simulink model "MIL_ASW"  (R2019b)
settings: Solver=FixedStepDiscrete  StartTime=0.0  StopTime=2  FixedStep=0.001  RelTol=1e-3  EnableMultiTasking=on
model workspace (MAT data in the model file):
  AccPedlCanVal : Simulink.Signal (value not decoded)
  AccPedlVal : Simulink.Signal (value not decoded)
  BrkPedlCanVal : Simulink.Signal (value not decoded)
  BrkPedlVal : Simulink.Signal (value not decoded)
  Cal1 : Simulink.Parameter (value not decoded)
  Cal10 : Simulink.Parameter (value not decoded)
  Cal11 : Simulink.Parameter (value not decoded)
  Cal12 : Simulink.Parameter (value not decoded)
  Cal2 : Simulink.Parameter (value not decoded)
  Cal3 : Simulink.Parameter (value not decoded)
  Cal4 : Simulink.Parameter (value not decoded)
  Cal5 : Simulink.Parameter (value not decoded)
  Cal6 : Simulink.Parameter (value not decoded)
  Cal7 : Simulink.Parameter (value not decoded)
  Cal8 : Simulink.Parameter (value not decoded)
  Cal9 : Simulink.Parameter (value not decoded)
  Clu1Act : Simulink.Signal (value not decoded)
  Clu1PTar : Simulink.Signal (value not decoded)
  Clu1Req : Simulink.Signal (value not decoded)
  Clu1TqTar : Simulink.Signal (value not decoded)
  Clu2Act : Simulink.Signal (value not decoded)
  Clu2PTar : Simulink.Signal (value not decoded)
  Clu2Req : Simulink.Signal (value not decoded)
  Clu2TqTar : Simulink.Signal (value not decoded)
  CluKissPtPLnch : Simulink.Parameter (value not decoded)
  CluOilTRawVal : Simulink.Signal (value not decoded)
  CluOilTVal : Simulink.Signal (value not decoded)
  CluOpenTqRatMax : Simulink.Parameter (value not decoded)
  CluPMap : Simulink.Parameter (value not decoded)
  CluPMax : Simulink.Parameter (value not decoded)
  CluPMaxGear1 : Simulink.Parameter (value not decoded)
  CluPMaxGear2 : Simulink.Parameter (value not decoded)
  CluPMaxGear3 : Simulink.Parameter (value not decoded)
  CluPMaxGear4 : Simulink.Parameter (value not decoded)
  CluPMaxGear5 : Simulink.Parameter (value not decoded)
  CluPMaxGear6 : Simulink.Parameter (value not decoded)
  CluPMaxGearR : Simulink.Parameter (value not decoded)
  CluPMin : Simulink.Parameter (value not decoded)
  CluPosnMax : Simulink.Parameter (value not decoded)
  CluSoln1IRawVal : Simulink.Signal (value not decoded)
  CluSoln1IReq : Simulink.Signal (value not decoded)
  CluSoln1IReqFlg : Simulink.Signal (value not decoded)
  CluSoln1IVal : Simulink.Signal (value not decoded)
  CluSoln1LineI : Simulink.Parameter (value not decoded)
  CluSoln1LineP : Simulink.Parameter (value not decoded)
  CluSoln1Pwm : Simulink.Signal (value not decoded)
  CluSoln2IRawVal : Simulink.Signal (value not decoded)
  CluSoln2IReq : Simulink.Signal (value not decoded)
  CluSoln2IReqFlg : Simulink.Signal (value not decoded)
  CluSoln2IVal : Simulink.Signal (value not decoded)
  CluSoln2LineI : Simulink.Parameter (value not decoded)
  CluSoln2LineP : Simulink.Parameter (value not decoded)
  CluSoln2Pwm : Simulink.Signal (value not decoded)
  CluTqMap : Simulink.Parameter (value not decoded)
  CrnkSpdRawVal : Simulink.Signal (value not decoded)
  CrnkSpdVal : Simulink.Signal (value not decoded)
  Drive_Intensity_Fuzzy : object (value not decoded)
  DrvIntenFzzy : Simulink.LookupTable (value not decoded)
  EngNIdle : Simulink.Parameter (value not decoded)
  EngNIdleMin : Simulink.Parameter (value not decoded)
  EngSpdCanVal : Simulink.Signal (value not decoded)
  EngThrCanVal : Simulink.Signal (value not decoded)
  EngTqAdd : Simulink.Parameter (value not decoded)
  EngTqCanVal : Simulink.Signal (value not decoded)
  EngTqIntvFlg : Simulink.Signal (value not decoded)
  EngTqIntvRat : Simulink.Signal (value not decoded)
  EngTqMapExtChartc : Simulink.Parameter (value not decoded)
  EngTqMapSpdIndx : Simulink.Parameter (value not decoded)
  EngTqMapThrtIndx : Simulink.Parameter (value not decoded)
  EngTqMapTqMax : Simulink.Parameter (value not decoded)
  EngTqMaxNorm : Simulink.Parameter (value not decoded)
  EngTqRef : Simulink.Parameter (value not decoded)
  EvenCluPRawVal : Simulink.Signal (value not decoded)
  EvenCluPVal : Simulink.Signal (value not decoded)
  EvenInpSpdRawVal : Simulink.Signal (value not decoded)
  EvenInpSpdVal : Simulink.Signal (value not decoded)
  FcnCallTime : Simulink.Parameter (value not decoded)
  FinalRat : Simulink.Parameter (value not decoded)
  Fork1A : Simulink.Parameter (value not decoded)
  Fork1Act : Simulink.Signal (value not decoded)
  Fork1B : Simulink.Parameter (value not decoded)
  Fork1DeltaSpdTar : Simulink.Parameter (value not decoded)
  Fork1MaxSpd1A : Simulink.Parameter (value not decoded)
  Fork1MaxSpd1B : Simulink.Parameter (value not decoded)
  Fork1MaxSpd2A : Simulink.Parameter (value not decoded)
  Fork1MaxSpd2B : Simulink.Parameter (value not decoded)
  Fork1PosnA : Simulink.Parameter (value not decoded)
  Fork1PosnB : Simulink.Parameter (value not decoded)
  Fork1PosnMaxSpd1A : Simulink.Parameter (value not decoded)
  Fork1PosnMaxSpd1B : Simulink.Parameter (value not decoded)
  Fork1PosnMaxSpd2A : Simulink.Parameter (value not decoded)
  Fork1PosnMaxSpd2B : Simulink.Parameter (value not decoded)
  Fork1PosnNeut : Simulink.Parameter (value not decoded)
  Fork1PosnNeutA : Simulink.Parameter (value not decoded)
  Fork1PosnNeutB : Simulink.Parameter (value not decoded)
  Fork1PosnRawVal : Simulink.Signal (value not decoded)
  Fork1PosnSyncA : Simulink.Parameter (value not decoded)
  Fork1PosnSyncB : Simulink.Parameter (value not decoded)
  Fork1PosnVal : Simulink.Signal (value not decoded)
  Fork1SyncTar : Simulink.Parameter (value not decoded)
  Fork2A : Simulink.Parameter (value not decoded)
  Fork2Act : Simulink.Signal (value not decoded)
  Fork2B : Simulink.Parameter (value not decoded)
  Fork2DeltaSpdTar : Simulink.Parameter (value not decoded)
  Fork2MaxSpd1A : Simulink.Parameter (value not decoded)
  Fork2MaxSpd1B : Simulink.Parameter (value not decoded)
  Fork2MaxSpd2A : Simulink.Parameter (value not decoded)
  Fork2MaxSpd2B : Simulink.Parameter (value not decoded)
  Fork2PosnA : Simulink.Parameter (value not decoded)
  Fork2PosnB : Simulink.Parameter (value not decoded)
  Fork2PosnMaxSpd1A : Simulink.Parameter (value not decoded)
  Fork2PosnMaxSpd1B : Simulink.Parameter (value not decoded)
  Fork2PosnMaxSpd2A : Simulink.Parameter (value not decoded)
  Fork2PosnMaxSpd2B : Simulink.Parameter (value not decoded)
  Fork2PosnNeut : Simulink.Parameter (value not decoded)
  Fork2PosnNeutA : Simulink.Parameter (value not decoded)
  Fork2PosnNeutB : Simulink.Parameter (value not decoded)
  Fork2PosnRawVal : Simulink.Signal (value not decoded)
  Fork2PosnSyncA : Simulink.Parameter (value not decoded)
  Fork2PosnSyncB : Simulink.Parameter (value not decoded)
  Fork2PosnVal : Simulink.Signal (value not decoded)
  Fork2SyncTar : Simulink.Parameter (value not decoded)
  Fork3A : Simulink.Parameter (value not decoded)
  Fork3Act : Simulink.Signal (value not decoded)
  Fork3B : Simulink.Parameter (value not decoded)
  Fork3DeltaSpdTar : Simulink.Parameter (value not decoded)
  Fork3MaxSpd1A : Simulink.Parameter (value not decoded)
  Fork3MaxSpd1B : Simulink.Parameter (value not decoded)
  Fork3MaxSpd2A : Simulink.Parameter (value not decoded)
  Fork3MaxSpd2B : Simulink.Parameter (value not decoded)
  Fork3PosnA : Simulink.Parameter (value not decoded)
  Fork3PosnB : Simulink.Parameter (value not decoded)
  Fork3PosnMaxSpd1A : Simulink.Parameter (value not decoded)
  Fork3PosnMaxSpd1B : Simulink.Parameter (value not decoded)
  Fork3PosnMaxSpd2A : Simulink.Parameter (value not decoded)
  Fork3PosnMaxSpd2B : Simulink.Parameter (value not decoded)
  Fork3PosnNeut : Simulink.Parameter (value not decoded)
  Fork3PosnNeutA : Simulink.Parameter (value not decoded)
  Fork3PosnNeutB : Simulink.Parameter (value not decoded)
  Fork3PosnRawVal : Simulink.Signal (value not decoded)
  Fork3PosnSyncA : Simulink.Parameter (value not decoded)
  Fork3PosnSyncB : Simulink.Parameter (value not decoded)
  Fork3PosnVal : Simulink.Signal (value not decoded)
  Fork3SyncTar : Simulink.Parameter (value not decoded)
  Fork4A : Simulink.Parameter (value not decoded)
  Fork4Act : Simulink.Signal (value not decoded)
  Fork4B : Simulink.Parameter (value not decoded)
  Fork4DeltaSpdTar : Simulink.Parameter (value not decoded)
  Fork4MaxSpd1A : Simulink.Parameter (value not decoded)
  Fork4MaxSpd1B : Simulink.Parameter (value not decoded)
  Fork4MaxSpd2A : Simulink.Parameter (value not decoded)
  Fork4MaxSpd2B : Simulink.Parameter (value not decoded)
  Fork4PosnA : Simulink.Parameter (value not decoded)
  Fork4PosnB : Simulink.Parameter (value not decoded)
  Fork4PosnMaxSpd1A : Simulink.Parameter (value not decoded)
  Fork4PosnMaxSpd1B : Simulink.Parameter (value not decoded)
  Fork4PosnMaxSpd2A : Simulink.Parameter (value not decoded)
  Fork4PosnMaxSpd2B : Simulink.Parameter (value not decoded)
  Fork4PosnNeut : Simulink.Parameter (value not decoded)
  Fork4PosnNeutA : Simulink.Parameter (value not decoded)
  Fork4PosnNeutB : Simulink.Parameter (value not decoded)
  Fork4PosnRawVal : Simulink.Signal (value not decoded)
  Fork4PosnSyncA : Simulink.Parameter (value not decoded)
  Fork4PosnSyncB : Simulink.Parameter (value not decoded)
  Fork4PosnVal : Simulink.Signal (value not decoded)
  Fork4SyncTar : Simulink.Parameter (value not decoded)
  FrntWhlRd : Simulink.Parameter (value not decoded)
  GearIdx : Simulink.Parameter (value not decoded)
  GearMax : Simulink.Parameter (value not decoded)
  GearRat : Simulink.Parameter (value not decoded)
  Launch_Engage_Fuzzy : object (value not decoded)
  LnchEngmtFzzy : Simulink.LookupTable (value not decoded)
  LubeSolnIRawVal : Simulink.Signal (value not decoded)
  LubeSolnIReq : Simulink.Signal (value not decoded)
  LubeSolnIVal : Simulink.Signal (value not decoded)
  LubeSolnLineI : Simulink.Parameter (value not decoded)
  LubeSolnLineP : Simulink.Parameter (value not decoded)
  LubeSolnPwm : Simulink.Signal (value not decoded)
  MaiLineSolnIRawVal : Simulink.Signal (value not decoded)
  MaiLineSolnIReq : Simulink.Signal (value not decoded)
  MaiLineSolnIVal : Simulink.Signal (value not decoded)
  MaiLineSolnLineI : Simulink.Parameter (value not decoded)
  MaiLineSolnLineP : Simulink.Parameter (value not decoded)
  MaiLineSolnPwm : Simulink.Signal (value not decoded)
  OddCluPRawVal : Simulink.Signal (value not decoded)
  OddCluPVal : Simulink.Signal (value not decoded)
  OddInpSpdRawVal : Simulink.Signal (value not decoded)
  OddInpSpdVal : Simulink.Signal (value not decoded)
  OutpSpdRawVal : Simulink.Signal (value not decoded)
  OutpSpdVal : Simulink.Signal (value not decoded)
  PsnsrLineP : Simulink.Parameter (value not decoded)
  PsnsrLineV : Simulink.Parameter (value not decoded)
  SftLvrCanVal : Simulink.Signal (value not decoded)
  SftLvrCfm : Simulink.Signal (value not decoded)
  SftLvrVal : Simulink.Signal (value not decoded)
  Shaft1GearAct : Simulink.Signal (value not decoded)
  Shaft1GearReq : Simulink.Signal (value not decoded)
  Shaft2GearAct : Simulink.Signal (value not decoded)
  Shaft2GearReq : Simulink.Signal (value not decoded)
  ShiftMux1SwtReq : Simulink.Signal (value not decoded)
  ShiftMux2SwtReq : Simulink.Signal (value not decoded)
  ShiftSdlEcoDwnSeln : Simulink.Parameter (value not decoded)
  ShiftSdlEcoDwnShift : Simulink.Parameter (value not decoded)
  ShiftSdlEcoUpSeln : Simulink.Parameter (value not decoded)
  ShiftSdlEcoUpShift : Simulink.Parameter (value not decoded)
  ShiftSdlPwrDwnSeln : Simulink.Parameter (value not decoded)
  ShiftSdlPwrDwnShift : Simulink.Parameter (value not decoded)
  ShiftSdlPwrUpSeln : Simulink.Parameter (value not decoded)
  ShiftSdlPwrUpShift : Simulink.Parameter (value not decoded)
  ShiftSdlSACDwnSeln : Simulink.Parameter (value not decoded)
  ShiftSdlSACDwnShift : Simulink.Parameter (value not decoded)
  ShiftSdlSACUpSeln : Simulink.Parameter (value not decoded)
  ShiftSdlSACUpShift : Simulink.Parameter (value not decoded)
  ShiftSdlThrPedlIdx : Simulink.Parameter (value not decoded)
  ShiftSoln1IRawVal : Simulink.Signal (value not decoded)
  ShiftSoln1IReq : Simulink.Signal (value not decoded)
  ShiftSoln1IVal : Simulink.Signal (value not decoded)
  ShiftSoln1LineI : Simulink.Parameter (value not decoded)
  ShiftSoln1LineP : Simulink.Parameter (value not decoded)
  ShiftSoln1Pwm : Simulink.Signal (value not decoded)
  ShiftSoln2IRawVal : Simulink.Signal (value not decoded)
  ShiftSoln2IReq : Simulink.Signal (value not decoded)
  ShiftSoln2IVal : Simulink.Signal (value not decoded)
  ShiftSoln2LineI : Simulink.Parameter (value not decoded)
  ShiftSoln2LineP : Simulink.Parameter (value not decoded)
  ShiftSoln2Pwm : Simulink.Signal (value not decoded)
  SolnOutpTRawVal : Simulink.Signal (value not decoded)
  SolnOutpTVal : Simulink.Signal (value not decoded)
  TSnsr1LineR : Simulink.Parameter (value not decoded)
  TSnsr2LineR : Simulink.Parameter (value not decoded)
  TrsmNrGearAct : Simulink.Signal (value not decoded)
  TrsmNrGearReq : Simulink.Signal (value not decoded)
  TrsmNrPreGearAct : Simulink.Signal (value not decoded)
  TrsmNrPreGearReq : Simulink.Signal (value not decoded)
  Tsnsr1LineT : Simulink.Parameter (value not decoded)
  Tsnsr2LineT : Simulink.Parameter (value not decoded)
  VehSpdCanVal : Simulink.Signal (value not decoded)
  VehSpdTrsmEstimd : Simulink.Signal (value not decoded)
  VehSpdVal : Simulink.Signal (value not decoded)
  VlvBodyTRawVal : Simulink.Signal (value not decoded)
  VlvBodyTVal : Simulink.Signal (value not decoded)
symbols that are objects in the model workspace (value not decoded): CluPMap, CluSoln1LineI, CluSoln1LineP, CluSoln2LineI, CluSoln2LineP, CluTqMap, EngNIdle, EngNIdleMin, EngTqMapThrtIndx, EngTqMapTqMax, EngTqMaxNorm, FcnCallTime, FinalRat, Fork1A, Fork1B, Fork1DeltaSpdTar, Fork1PosnA, Fork1PosnB, Fork1PosnMaxSpd1A, Fork1PosnMaxSpd1B, Fork1PosnMaxSpd2A, Fork1PosnMaxSpd2B, Fork1PosnNeut, Fork1PosnNeutA, Fork1PosnNeutB, Fork1PosnSyncA, Fork1PosnSyncB, Fork1SyncTar, Fork2A, Fork2B, Fork2DeltaSpdTar, Fork2PosnA, Fork2PosnB, Fork2PosnMaxSpd1A, Fork2PosnMaxSpd1B, Fork2PosnMaxSpd2A, Fork2PosnMaxSpd2B, Fork2PosnNeut, Fork2PosnNeutA, Fork2PosnNeutB, Fork2PosnSyncA, Fork2PosnSyncB, Fork2SyncTar, Fork3A, Fork3B, Fork3DeltaSpdTar, Fork3PosnA, Fork3PosnB, Fork3PosnMaxSpd1A, Fork3PosnMaxSpd1B, Fork3PosnMaxSpd2A, Fork3PosnMaxSpd2B, Fork3PosnNeut, Fork3PosnNeutA, Fork3PosnNeutB, Fork3PosnSyncA, Fork3PosnSyncB, Fork3SyncTar, Fork4A, Fork4B
undefined symbols (not defined in the file or in its folder): in1, out1
libraries: simulink x44, fuzblock x3
(part 5 of 10)

== system MIL_ASW/Application_Software_SHAW/ASW_GearPressureControl/Fork 3 ==
  ForkDirReq : Inport
  ForkSyncPha : Inport  Port=2
  ForkDeltaSpdReq : Inport  Port=3
  ForkPosnReq : Inport  Port=4
  ForkDeltaSpdAct : Inport  Port=5
  ForkPosnVal : Inport  Port=6
  Enable : EnablePort  StatesWhenEnabling=reset
  Abs : Abs  OutDataTypeStr=uint16
  Abs2 : Abs  OutDataTypeStr=uint16
  Add4 : Sum  Inputs=+-  OutDataTypeStr=int16
  Add6 : Sum  Inputs=+-  OutDataTypeStr=int16
  Compare To Constant : simulink/Logic and Bit Operations/Compare To Constant  relop===  const=2  OutDataTypeStr=boolean
  Compare To Constant1 : simulink/Logic and Bit Operations/Compare To Constant  relop===  const=1  OutDataTypeStr=boolean
  Compare To Constant2 : simulink/Logic and Bit Operations/Compare To Constant  relop===  const=3  OutDataTypeStr=boolean
  Compare To Constant3 : simulink/Logic and Bit Operations/Compare To Constant  relop===  const=2  OutDataTypeStr=boolean
  Compare To Constant4 : simulink/Logic and Bit Operations/Compare To Constant  relop===  const=4  OutDataTypeStr=boolean
  Constant : Constant  Value=150  OutDataTypeStr=uint16
  Gain : Gain  Gain=5  OutDataTypeStr=uint16
  Gain1 : Gain  OutDataTypeStr=uint16
  Logical Operator : Logic  Operator=OR  AllPortsSameDT=off  OutDataTypeStr=boolean
  Logical Operator1 : Logic  Operator=OR  AllPortsSameDT=off  OutDataTypeStr=boolean
  Saturation : Saturate  UpperLimit=300  LowerLimit=0  OutDataTypeStr=uint16
  Switch : Switch  Criteria=u2 > Threshold
  Switch1 : Switch  Criteria=u2 > Threshold
  Switch2 : Switch  Criteria=u2 > Threshold
  Terminator : Terminator
  ForkPReq : Outport  VectorParamsAs1DForOutWhenUnconnected=off
  wires:
  ForkPosnReq/1 -> Switch1/1, Switch2/1
  ForkDeltaSpdReq/1 -> Add6/1
  ForkDeltaSpdAct/1 -> Add6/2
  Add6/1 -> Abs2/1
  Add4/1 -> Abs/1
  Abs2/1 -> Gain1/1
  Compare To Constant/1 -> Switch/2
  ForkSyncPha/1 -> Compare To Constant/1
  Constant/1 -> Switch/1
  Gain/1 -> Switch/3
  ForkDirReq/1 -> Compare To Constant3/1, Compare To Constant1/1, Compare To Constant4/1, Compare To Constant2/1
  Compare To Constant1/1 -> Logical Operator/1
  Compare To Constant3/1 -> Logical Operator/2
  Compare To Constant2/1 -> Logical Operator1/1
  Compare To Constant4/1 -> Logical Operator1/2
  Logical Operator/1 -> Switch1/2
  ForkPosnVal/1 -> Switch2/3, Switch1/3
  Logical Operator1/1 -> Switch2/2
  Switch1/1 -> Add4/1
  Switch2/1 -> Add4/2
  Switch/1 -> Saturation/1
  Saturation/1 -> ForkPReq/1
  Gain1/1 -> Terminator/1
  Abs/1 -> Gain/1

== system MIL_ASW/Application_Software_SHAW/ASW_GearPressureControl/Fork 4 ==
  ForkDirReq : Inport
  ForkSyncPha : Inport  Port=2
  ForkDeltaSpdReq : Inport  Port=3
  ForkPosnReq : Inport  Port=4
  ForkDeltaSpdAct : Inport  Port=5
  ForkPosnVal : Inport  Port=6
  Enable : EnablePort  StatesWhenEnabling=reset
  Abs : Abs  OutDataTypeStr=uint16
  Abs2 : Abs  OutDataTypeStr=uint16
  Add4 : Sum  Inputs=+-  OutDataTypeStr=int16
  Add6 : Sum  Inputs=+-  OutDataTypeStr=int16
  Compare To Constant : simulink/Logic and Bit Operations/Compare To Constant  relop===  const=2  OutDataTypeStr=boolean
  Compare To Constant1 : simulink/Logic and Bit Operations/Compare To Constant  relop===  const=1  OutDataTypeStr=boolean
  Compare To Constant2 : simulink/Logic and Bit Operations/Compare To Constant  relop===  const=3  OutDataTypeStr=boolean
  Compare To Constant3 : simulink/Logic and Bit Operations/Compare To Constant  relop===  const=2  OutDataTypeStr=boolean
  Compare To Constant4 : simulink/Logic and Bit Operations/Compare To Constant  relop===  const=4  OutDataTypeStr=boolean
  Constant : Constant  Value=150  OutDataTypeStr=uint16
  Gain : Gain  Gain=5  OutDataTypeStr=uint16
  Gain1 : Gain  OutDataTypeStr=uint16
  Logical Operator : Logic  Operator=OR  AllPortsSameDT=off  OutDataTypeStr=boolean
  Logical Operator1 : Logic  Operator=OR  AllPortsSameDT=off  OutDataTypeStr=boolean
  Saturation : Saturate  UpperLimit=300  LowerLimit=0  OutDataTypeStr=uint16
  Switch : Switch  Criteria=u2 > Threshold
  Switch1 : Switch  Criteria=u2 > Threshold
  Switch2 : Switch  Criteria=u2 > Threshold
  Terminator : Terminator
  ForkPReq : Outport  VectorParamsAs1DForOutWhenUnconnected=off
  wires:
  Abs/1 -> Gain/1
  Gain1/1 -> Terminator/1
  Saturation/1 -> ForkPReq/1
  Switch/1 -> Saturation/1
  Switch2/1 -> Add4/2
  Switch1/1 -> Add4/1
  Logical Operator1/1 -> Switch2/2
  ForkPosnVal/1 -> Switch1/3, Switch2/3
  Logical Operator/1 -> Switch1/2
  Compare To Constant4/1 -> Logical Operator1/2
  Compare To Constant2/1 -> Logical Operator1/1
  Compare To Constant3/1 -> Logical Operator/2
  Compare To Constant1/1 -> Logical Operator/1
  ForkDirReq/1 -> Compare To Constant2/1, Compare To Constant4/1, Compare To Constant1/1, Compare To Constant3/1
  Gain/1 -> Switch/3
  Constant/1 -> Switch/1
  ForkSyncPha/1 -> Compare To Constant/1
  Compare To Constant/1 -> Switch/2
  Abs2/1 -> Gain1/1
  Add4/1 -> Abs/1
  Add6/1 -> Abs2/1
  ForkDeltaSpdAct/1 -> Add6/2
  ForkDeltaSpdReq/1 -> Add6/1
  ForkPosnReq/1 -> Switch2/1, Switch1/1

== system MIL_ASW/Application_Software_SHAW/ASW_GearPressureControl/PID ==
  In1 : Inport
  1/100 : Gain  Gain=1/100  OutDataTypeStr=uint16
  1/1000ms : Gain  Gain=1/1000  OutDataTypeStr=int32
  Add1 : Sum  Inputs=+-+  OutDataTypeStr=int16
  Add7 : Sum  Inputs=+-  OutDataTypeStr=int16
  Add8 : Sum  Inputs=+++  OutDataTypeStr=int32
  Add9 : Sum  OutDataTypeStr=int32
  Gain2 : Gain  Gain=1000/FcnCallTime  OutDataTypeStr=int32
  Gain3 : Gain  Gain=FcnCallTime  OutDataTypeStr=int32
  Gain4 : Gain  Gain=1000  OutDataTypeStr=int32
  Gain6 : Gain  Gain=2  OutDataTypeStr=int32
  Kd*100 : Gain  Gain=0  OutDataTypeStr=int32
  Ki*100 : Gain  Gain=100  OutDataTypeStr=int32
  Kp*100 : Gain  Gain=15  OutDataTypeStr=int32
  Memory{1..3,5} (4 alike) : Memory  InheritSampleTime=on
  Saturation1 : Saturate  UpperLimit=100000  LowerLimit=0  OutDataTypeStr=int32
  Saturation2 : Saturate  UpperLimit=30000  LowerLimit=-30000
  Out1 : Outport  VectorParamsAs1DForOutWhenUnconnected=off
  wires:
  Add7/1 -> Kp*100/1
  Saturation2/1 -> Add9/2
  Ki*100/1 -> Gain3/1
  Kp*100/1 -> Gain4/1
  Memory2/1 -> Add7/2
  Saturation1/1 -> 1/100/1, Memory3/1
  Add9/1 -> Saturation1/1
  Add8/1 -> 1/1000ms/1
  In1/1 -> Add7/1, Memory1/1, Add1/1, Ki*100/1, Memory2/1
  Gain3/1 -> Add8/2
  Gain4/1 -> Add8/1
  Memory3/1 -> Add9/1
  Add1/1 -> Kd*100/1
  Gain6/1 -> Add1/2
  Kd*100/1 -> Gain2/1
  Memory5/1 -> Add1/3
  Gain2/1 -> Add8/3
  Memory1/1 -> Memory5/1, Gain6/1
  1/1000ms/1 -> Saturation2/1
  1/100/1 -> Out1/1

== system MIL_ASW/Application_Software_SHAW/ASW_GearPressureControl/PID1 ==
  In1 : Inport
  1/100 : Gain  Gain=1/100  OutDataTypeStr=uint16
  1/1000ms : Gain  Gain=1/1000  OutDataTypeStr=int32
  Add1 : Sum  Inputs=+-+  OutDataTypeStr=int16
  Add7 : Sum  Inputs=+-  OutDataTypeStr=int16
  Add8 : Sum  Inputs=+++  OutDataTypeStr=int32
  Add9 : Sum  OutDataTypeStr=int32
  Gain2 : Gain  Gain=1000/FcnCallTime  OutDataTypeStr=int32
  Gain3 : Gain  Gain=FcnCallTime  OutDataTypeStr=int32
  Gain4 : Gain  Gain=1000  OutDataTypeStr=int32
  Gain6 : Gain  Gain=2  OutDataTypeStr=int32
  Kd*100 : Gain  Gain=0  OutDataTypeStr=int32
  Ki*100 : Gain  Gain=100  OutDataTypeStr=int32
  Kp*100 : Gain  Gain=15  OutDataTypeStr=int32
  Memory{1..3,5} (4 alike) : Memory  InheritSampleTime=on
  Saturation1 : Saturate  UpperLimit=100000  LowerLimit=0  OutDataTypeStr=int32
  Saturation2 : Saturate  UpperLimit=30000  LowerLimit=-30000
  Out1 : Outport  VectorParamsAs1DForOutWhenUnconnected=off
  wires:
  1/100/1 -> Out1/1
  1/1000ms/1 -> Saturation2/1
  Memory1/1 -> Gain6/1, Memory5/1
  Gain2/1 -> Add8/3
  Memory5/1 -> Add1/3
  Kd*100/1 -> Gain2/1
  Gain6/1 -> Add1/2
  Add1/1 -> Kd*100/1
  Memory3/1 -> Add9/1
  Gain4/1 -> Add8/1
  Gain3/1 -> Add8/2
  In1/1 -> Memory2/1, Ki*100/1, Add1/1, Memory1/1, Add7/1
  Add8/1 -> 1/1000ms/1
  Add9/1 -> Saturation1/1
  Saturation1/1 -> Memory3/1, 1/100/1
  Memory2/1 -> Add7/2
  Kp*100/1 -> Gain4/1
  Ki*100/1 -> Gain3/1
  Saturation2/1 -> Add9/2
  Add7/1 -> Kp*100/1

== system MIL_ASW/Application_Software_SHAW/ASW_Interface/Accelerator Pedal Value Process ==
  AccPedlCanVal : Inport
  BrkPedlVal : Inport  Port=2
  Constant : Constant  Value=0  OutDataTypeStr=uint8
  Gain : Gain  Gain=100/255  OutDataTypeStr=uint8
  Switch : Switch  Criteria=u2 > Threshold  OutDataTypeStr=uint8
  AccPedlVal : Outport  OutDataTypeStr=uint8  VectorParamsAs1DForOutWhenUnconnected=off
  wires:
  BrkPedlVal/1 -> Switch/2
  Switch/1 -> Gain/1
  Constant/1 -> Switch/1
  Gain/1 -> AccPedlVal/1
  AccPedlCanVal/1 -> Switch/3

== system MIL_ASW/Application_Software_SHAW/ASW_Interface/Brake Pedal Value Process ==
  BrkPedlCanVal : Inport
  Compare To Constant : simulink/Logic and Bit Operations/Compare To Constant  relop=>  const=30  OutDataTypeStr=uint8
  Gain : Gain  Gain=100/255  OutDataTypeStr=uint8
  BrkPedlVal : Outport  OutDataTypeStr=uint8  VectorParamsAs1DForOutWhenUnconnected=off
  BrkSig : Outport  Port=2  OutDataTypeStr=uint8  VectorParamsAs1DForOutWhenUnconnected=off
  wires:
  Gain/1 -> Compare To Constant/1, BrkPedlVal/1
  BrkPedlCanVal/1 -> Gain/1
  Compare To Constant/1 -> BrkSig/1

== system MIL_ASW/Application_Software_SHAW/ASW_Interface/Clutch Pressure Sensor Value Process ==
  OddCluPRawVal : Inport
  EvenCluPRawVal : Inport  Port=2
  1-D Lookup Table1 : Lookup_n-D  NumberOfTableDimensions=1  BreakpointsForDimension1=PsnsrLineV  Table=PsnsrLineP  TableDataTypeStr=Inherit: Inherit from 'Table data'  ExtrapMethod=Clip  UseLastTableValue=on  InternalRulePriority=Speed  OutDataTypeStr=Inherit: Inherit from 'Table data'  RndMeth=Simplest  InputSameDT=on
  1-D Lookup Table3 : Lookup_n-D  NumberOfTableDimensions=1  BreakpointsForDimension1=PsnsrLineV  Table=PsnsrLineP  TableDataTypeStr=Inherit: Inherit from 'Table data'  ExtrapMethod=Clip  UseLastTableValue=on  InternalRulePriority=Speed  OutDataTypeStr=Inherit: Inherit from 'Table data'  RndMeth=Simplest  InputSameDT=on
  Constant1 : Constant  Value=1023  OutDataTypeStr=uint16
  Constant2 : Constant  Value=1023  OutDataTypeStr=uint16
  Divide1 : Product  Inputs=*/  OutDataTypeStr=uint16
  Divide3 : Product  Inputs=*/  OutDataTypeStr=uint16
  Gain1 : Gain  Gain=5000  OutDataTypeStr=uint32
  Gain4 : Gain  Gain=5000  OutDataTypeStr=uint32
  OddCluPVal : Outport  VectorParamsAs1DForOutWhenUnconnected=off
  EvenCluPVal : Outport  Port=2  VectorParamsAs1DForOutWhenUnconnected=off
  wires:
  EvenCluPRawVal/1 -> Gain1/1
  1-D Lookup Table1/1 -> EvenCluPVal/1
  Gain4/1 -> Divide3/1
  Divide3/1 -> 1-D Lookup Table3/1  "mV"
  OddCluPRawVal/1 -> Gain4/1
  1-D Lookup Table3/1 -> OddCluPVal/1
  Constant2/1 -> Divide3/2
  Gain1/1 -> Divide1/1
  Divide1/1 -> 1-D Lookup Table1/1  "mV"
  Constant1/1 -> Divide1/2

== system MIL_ASW/Application_Software_SHAW/ASW_Interface/Engine Information from CAN bus ==
  EngThrCanVal : Inport
  EngSpdCanVal : Inport  Port=2
  EngTqCanVal : Inport  Port=3  OutDataTypeStr=uint16
  Constant : Constant  Value=84800  OutDataTypeStr=int32
  Constant1 : Constant  Value=0  OutDataTypeStr=int32
  Data Type Conversion : DataTypeConversion  OutDataTypeStr=uint16
  Gain : Gain  Gain=100/255  OutDataTypeStr=uint8
  Gain1 : Gain  Gain=1/4  ParamDataTypeStr=uint16  OutDataTypeStr=uint16
  Gain4 : Gain  Gain=100/2  OutDataTypeStr=int32
  MinMax : MinMax  Function=max  Inputs=2
  Subtract : Sum  Inputs=+-  OutDataTypeStr=int32
  EngThrVal : Outport  VectorParamsAs1DForOutWhenUnconnected=off
  EngSpdVal : Outport  Port=2  VectorParamsAs1DForOutWhenUnconnected=off
  EngTqVal : Outport  Port=3  VectorParamsAs1DForOutWhenUnconnected=off
  wires:
  EngSpdCanVal/1 -> Gain1/1
  EngTqCanVal/1 -> Gain4/1
  Gain4/1 -> Subtract/1
  EngThrCanVal/1 -> Gain/1
  Gain/1 -> EngThrVal/1
  Gain1/1 -> EngSpdVal/1
  Subtract/1 -> MinMax/1
  Constant/1 -> Subtract/2
  MinMax/1 -> Data Type Conversion/1
  Data Type Conversion/1 -> EngTqVal/1
  Constant1/1 -> MinMax/2

== system MIL_ASW/Application_Software_SHAW/ASW_Interface/Fork Position Sensor Value Process ==
  Fork1PosnRawVal : Inport
  Fork2PosnRawVal : Inport  Port=2
  Fork3PosnRawVal : Inport  Port=3
  Fork4PosnRawVal : Inport  Port=4
  Gain{1..4} (4 alike) : Gain  OutDataTypeStr=uint16
  Saturation{,1..3} (4 alike) : Saturate  UpperLimit=900  LowerLimit=100
  Fork1PosnVal : Outport  OutDataTypeStr=uint16  VectorParamsAs1DForOutWhenUnconnected=off
  Fork2PosnVal : Outport  Port=2  OutDataTypeStr=uint16  VectorParamsAs1DForOutWhenUnconnected=off
  Fork3PosnVal : Outport  Port=3  OutDataTypeStr=uint16  VectorParamsAs1DForOutWhenUnconnected=off
  Fork4PosnVal : Outport  Port=4  OutDataTypeStr=uint16  VectorParamsAs1DForOutWhenUnconnected=off
  wires:
  Fork1PosnRawVal/1 -> Gain4/1
  Gain4/1 -> Saturation/1
  Fork2PosnRawVal/1 -> Gain1/1
  Gain1/1 -> Saturation1/1
  Fork3PosnRawVal/1 -> Gain2/1
  Gain2/1 -> Saturation2/1
  Fork4PosnRawVal/1 -> Gain3/1
  Gain3/1 -> Saturation3/1
  Saturation/1 -> Fork1PosnVal/1
  Saturation1/1 -> Fork2PosnVal/1
  Saturation2/1 -> Fork3PosnVal/1
  Saturation3/1 -> Fork4PosnVal/1

== system MIL_ASW/Application_Software_SHAW/ASW_Interface/Shift Lever Value Process ==
  SftLvrCanVal : Inport
  Constant : Constant  Value=0  OutDataTypeStr=uint8
  Constant1 : Constant  OutDataTypeStr=uint8
  Constant2 : Constant  Value=2  OutDataTypeStr=uint8
  Constant3 : Constant  Value=3  OutDataTypeStr=uint8
  Constant4 : Constant  Value=2  OutDataTypeStr=uint8
  Multiport Switch : MultiPortSwitch  DataPortOrder=Specify indices  DataPortIndices={8,7,6,5}  DataPortForDefault=Additional data port  DiagnosticForDefault=Warning  OutDataTypeStr=uint8
  SftLvrVal : Outport  OutDataTypeStr=uint8  VectorParamsAs1DForOutWhenUnconnected=off
  wires:
  SftLvrCanVal/1 -> Multiport Switch/1
  Constant/1 -> Multiport Switch/2
  Constant1/1 -> Multiport Switch/3
  Constant2/1 -> Multiport Switch/4
  Constant3/1 -> Multiport Switch/5
  Constant4/1 -> Multiport Switch/6
  Multiport Switch/1 -> SftLvrVal/1

== system MIL_ASW/Application_Software_SHAW/ASW_Interface/Solenoid Current Value Process ==
  ShiftSoln1IRawVal : Inport
  ShiftSoln2IRawVal : Inport  Port=2
  MaiLineSolnIRawVal : Inport  Port=3
  LubeSolnIRawVal : Inport  Port=4
  CluSoln1IRawVal : Inport  Port=5
  CluSoln2IRawVal : Inport  Port=6
  Gain{,1..5} (6 alike) : Gain  Gain=1000/2*5/1023  OutDataTypeStr=uint16
  ShiftSoln1IVal : Outport  VectorParamsAs1DForOutWhenUnconnected=off
  ShiftSoln2IVal : Outport  Port=2  VectorParamsAs1DForOutWhenUnconnected=off
  MaiLineSolnIVal : Outport  Port=3  VectorParamsAs1DForOutWhenUnconnected=off
  LubeSolnIVal : Outport  Port=4  VectorParamsAs1DForOutWhenUnconnected=off
  CluSoln1IVal : Outport  Port=5  VectorParamsAs1DForOutWhenUnconnected=off
  CluSoln2IVal : Outport  Port=6  VectorParamsAs1DForOutWhenUnconnected=off
  wires:
  ShiftSoln1IRawVal/1 -> Gain/1
  Gain/1 -> ShiftSoln1IVal/1
  ShiftSoln2IRawVal/1 -> Gain1/1
  Gain1/1 -> ShiftSoln2IVal/1
  MaiLineSolnIRawVal/1 -> Gain2/1
  Gain2/1 -> MaiLineSolnIVal/1
  LubeSolnIRawVal/1 -> Gain3/1
  Gain3/1 -> LubeSolnIVal/1
  CluSoln1IRawVal/1 -> Gain4/1
  Gain4/1 -> CluSoln1IVal/1
  Gain5/1 -> CluSoln2IVal/1
  CluSoln2IRawVal/1 -> Gain5/1

== system MIL_ASW/Application_Software_SHAW/ASW_Interface/Speed Sensor Value Process ==
  CrnkSpdRawVal : Inport
  OddInpSpdRawVal : Inport  Port=2
  EvenInpSpdRawVal : Inport  Port=3
  OutpSpdRawVal : Inport  Port=4
  Constant : Constant  Value=2*314/100*FrntWhlRd/60*36/10  OutDataTypeStr=uint16
  Constant4 : Constant  Value=FinalRat(1)  OutDataTypeStr=uint16
  Divide4 : Product  Inputs=*/  OutDataTypeStr=uint16
  Gain : Gain  Gain=60/36  OutDataTypeStr=uint16
  Gain1 : Gain  Gain=60/36  OutDataTypeStr=uint16
  Gain2 : Gain  Gain=60/36  OutDataTypeStr=uint16
  Gain3 : Gain  Gain=60/18  OutDataTypeStr=uint16
  Gain4 : Gain  Gain=100  ParamDataTypeStr=uint16
  Product : Product  OutDataTypeStr=uint16
  Saturation : Saturate  UpperLimit=6800  LowerLimit=0
  Saturation1 : Saturate  UpperLimit=6800  LowerLimit=0
  Saturation2 : Saturate  UpperLimit=6800  LowerLimit=0
  Saturation3 : Saturate  UpperLimit=8940  LowerLimit=0
  CrnkSpdVal : Outport  VectorParamsAs1DForOutWhenUnconnected=off
  OddInpSpdVal : Outport  Port=2  VectorParamsAs1DForOutWhenUnconnected=off
  EvenInpSpdVal : Outport  Port=3  VectorParamsAs1DForOutWhenUnconnected=off
  OutpSpdVal : Outport  Port=4  VectorParamsAs1DForOutWhenUnconnected=off
  VehSpdTrsmEstimd : Outport  Port=5  VectorParamsAs1DForOutWhenUnconnected=off
  wires:
  CrnkSpdRawVal/1 -> Gain/1
  Gain/1 -> Saturation/1
  OddInpSpdRawVal/1 -> Gain1/1
  Gain1/1 -> Saturation1/1
  EvenInpSpdRawVal/1 -> Gain2/1
  Gain2/1 -> Saturation2/1
  OutpSpdRawVal/1 -> Gain3/1
  Divide4/1 -> Saturation3/1, Product/1
  Constant/1 -> Product/2
  Product/1 -> VehSpdTrsmEstimd/1
  Saturation/1 -> CrnkSpdVal/1
  Saturation1/1 -> OddInpSpdVal/1
  Saturation2/1 -> EvenInpSpdVal/1
  Saturation3/1 -> OutpSpdVal/1
  Constant4/1 -> Divide4/2
  Gain4/1 -> Divide4/1
  Gain3/1 -> Gain4/1

== system MIL_ASW/Application_Software_SHAW/ASW_Interface/Temperature Sensor Value Process ==
  CluOilTVal : Inport
  ValvBodyTRawVal : Inport  Port=2
  SolnOutpTRawVal : Inport  Port=3
  1-D Lookup Table1 : Lookup_n-D  NumberOfTableDimensions=1  BreakpointsForDimension1=TSnsr1LineR  Table=Tsnsr1LineT  TableDataTypeStr=Inherit: Inherit from 'Table data'  ExtrapMethod=Clip  UseLastTableValue=on  InternalRulePriority=Speed  OutDataTypeStr=Inherit: Inherit from 'Table data'  RndMeth=Simplest  InputSameDT=on
  1-D Lookup Table2 : Lookup_n-D  NumberOfTableDimensions=1  BreakpointsForDimension1=TSnsr2LineR  Table=Tsnsr2LineT  TableDataTypeStr=Inherit: Inherit from 'Table data'  ExtrapMethod=Clip  UseLastTableValue=on  InternalRulePriority=Speed  OutDataTypeStr=Inherit: Inherit from 'Table data'  RndMeth=Simplest  InputSameDT=on
  1-D Lookup Table3 : Lookup_n-D  NumberOfTableDimensions=1  BreakpointsForDimension1=TSnsr1LineR  Table=Tsnsr1LineT  TableDataTypeStr=Inherit: Inherit from 'Table data'  ExtrapMethod=Clip  UseLastTableValue=on  InternalRulePriority=Speed  OutDataTypeStr=Inherit: Inherit from 'Table data'  RndMeth=Simplest  InputSameDT=on
  Add1 : Sum  Inputs=-+
  Add2 : Sum  Inputs=-+
  Add3 : Sum  Inputs=-+
  Constant1 : Constant  Value=1023  OutDataTypeStr=uint16
  Constant2 : Constant  Value=1023  OutDataTypeStr=uint16
  Constant3 : Constant  Value=1023  OutDataTypeStr=uint16
  Divide1 : Product  Inputs=*/  OutDataTypeStr=uint16
  Divide2 : Product  Inputs=*/  OutDataTypeStr=uint16
  Divide3 : Product  Inputs=*/  OutDataTypeStr=uint16
  Gain : Gain  Gain=2600  OutDataTypeStr=uint32
  Gain1 : Gain  Gain=510  OutDataTypeStr=uint32
  Gain2 : Gain  Gain=2600  OutDataTypeStr=uint32
  CluOilTRawVal : Outport  VectorParamsAs1DForOutWhenUnconnected=off
  ValvBodyTVal : Outport  Port=2  VectorParamsAs1DForOutWhenUnconnected=off
  SolnOutpTVal : Outport  Port=3  VectorParamsAs1DForOutWhenUnconnected=off
  wires:
  Gain/1 -> Divide3/1
  Constant1/1 -> Add3/2
  Add3/1 -> Divide3/2
  Divide3/1 -> 1-D Lookup Table3/1  "R"
  CluOilTVal/1 -> Add3/1, Gain/1
  1-D Lookup Table3/1 -> CluOilTRawVal/1
  Divide2/1 -> 1-D Lookup Table2/1  "10R"
  1-D Lookup Table2/1 -> SolnOutpTVal/1
  Gain2/1 -> Divide1/1
  Constant3/1 -> Add2/2
  Add2/1 -> Divide1/2
  Divide1/1 -> 1-D Lookup Table1/1  "R"
  ValvBodyTRawVal/1 -> Gain2/1, Add2/1
  1-D Lookup Table1/1 -> ValvBodyTVal/1
  Gain1/1 -> Divide2/1
  Constant2/1 -> Add1/2
  Add1/1 -> Divide2/2
  SolnOutpTRawVal/1 -> Add1/1, Gain1/1

== system MIL_ASW/Application_Software_SHAW/ASW_Interface/Vehicle Speed Value Process ==
  VehSpdCanVal : Inport
  Gain : Gain  Gain=100/64  OutDataTypeStr=uint16
  VehSpdVal : Outport  VectorParamsAs1DForOutWhenUnconnected=off
  wires:
  VehSpdCanVal/1 -> Gain/1
  Gain/1 -> VehSpdVal/1

== system MIL_ASW/Application_Software_SHAW/ASW_MainLineControl/PID ==
  In1 : Inport
  1/100 : Gain  Gain=1/100  OutDataTypeStr=uint16
  1/1000ms : Gain  Gain=1/1000  OutDataTypeStr=int32
  Add1 : Sum  Inputs=+-+  OutDataTypeStr=int16
  Add7 : Sum  Inputs=+-  OutDataTypeStr=int16
  Add8 : Sum  Inputs=+++  OutDataTypeStr=int32
  Add9 : Sum  OutDataTypeStr=int32
  Gain2 : Gain  Gain=1000/FcnCallTime  OutDataTypeStr=int32
  Gain3 : Gain  Gain=FcnCallTime  OutDataTypeStr=int32
  Gain4 : Gain  Gain=1000  OutDataTypeStr=int32
  Gain6 : Gain  Gain=2  OutDataTypeStr=int32
  Kd*100 : Gain  Gain=0  OutDataTypeStr=int32
  Ki*100 : Gain  Gain=100  OutDataTypeStr=int32
  Kp*100 : Gain  Gain=15  OutDataTypeStr=int32
  Memory{1..3,5} (4 alike) : Memory  InheritSampleTime=on
  Saturation1 : Saturate  UpperLimit=100000  LowerLimit=0  OutDataTypeStr=int32
  Saturation2 : Saturate  UpperLimit=30000  LowerLimit=-30000
  Out1 : Outport  VectorParamsAs1DForOutWhenUnconnected=off
  wires:
  Add7/1 -> Kp*100/1
  Saturation2/1 -> Add9/2
  Ki*100/1 -> Gain3/1
  Kp*100/1 -> Gain4/1
  Memory2/1 -> Add7/2
  Saturation1/1 -> 1/100/1, Memory3/1
  Add9/1 -> Saturation1/1
  Add8/1 -> 1/1000ms/1
  In1/1 -> Add7/1, Memory1/1, Add1/1, Ki*100/1, Memory2/1
  Gain3/1 -> Add8/2
  Gain4/1 -> Add8/1
  Memory3/1 -> Add9/1
  Add1/1 -> Kd*100/1
  Gain6/1 -> Add1/2
  Kd*100/1 -> Gain2/1
  Memory5/1 -> Add1/3
  Gain2/1 -> Add8/3
  Memory1/1 -> Memory5/1, Gain6/1
  1/1000ms/1 -> Saturation2/1
  1/100/1 -> Out1/1

== system MIL_ASW/Application_Software_SHAW/ASW_MainLineControl/PID1 ==
  In1 : Inport
  1/100 : Gain  Gain=1/100  OutDataTypeStr=uint16
  1/1000ms : Gain  Gain=1/1000  OutDataTypeStr=int32
  Add1 : Sum  Inputs=+-+  OutDataTypeStr=int16
  Add7 : Sum  Inputs=+-  OutDataTypeStr=int16
  Add8 : Sum  Inputs=+++  OutDataTypeStr=int32
  Add9 : Sum  OutDataTypeStr=int32
  Gain2 : Gain  Gain=1000/FcnCallTime  OutDataTypeStr=int32
  Gain3 : Gain  Gain=FcnCallTime  OutDataTypeStr=int32
  Gain4 : Gain  Gain=1000  OutDataTypeStr=int32
  Gain6 : Gain  Gain=2  OutDataTypeStr=int32
  Kd*100 : Gain  Gain=0  OutDataTypeStr=int32
  Ki*100 : Gain  Gain=100  OutDataTypeStr=int32
  Kp*100 : Gain  Gain=15  OutDataTypeStr=int32
  Memory{1..3,5} (4 alike) : Memory  InheritSampleTime=on
  Saturation1 : Saturate  UpperLimit=100000  LowerLimit=0  OutDataTypeStr=int32
  Saturation2 : Saturate  UpperLimit=30000  LowerLimit=-30000
  Out1 : Outport  VectorParamsAs1DForOutWhenUnconnected=off
  wires:
  Add7/1 -> Kp*100/1
  Saturation2/1 -> Add9/2
  Ki*100/1 -> Gain3/1
  Kp*100/1 -> Gain4/1
  Memory2/1 -> Add7/2
  Saturation1/1 -> 1/100/1, Memory3/1
  Add9/1 -> Saturation1/1
  Add8/1 -> 1/1000ms/1
  In1/1 -> Add7/1, Memory1/1, Add1/1, Ki*100/1, Memory2/1
  Gain3/1 -> Add8/2
  Gain4/1 -> Add8/1
  Memory3/1 -> Add9/1
  Add1/1 -> Kd*100/1
  Gain6/1 -> Add1/2
  Kd*100/1 -> Gain2/1
  Memory5/1 -> Add1/3
  Gain2/1 -> Add8/3
  Memory1/1 -> Memory5/1, Gain6/1
  1/1000ms/1 -> Saturation2/1
  1/100/1 -> Out1/1

== system MIL_ASW/Application_Software_SHAW/ASW_ShaftAccessControl/Shift lever match to gear ==
  SftLvrVal : Inport
  TrsmNrGearAct : Inport  Port=2
  TrsmNrPreGearAct : Inport  Port=3
  Shift lever confirm logic : Stateflow chart  TreatAsAtomicUnit=on
  SftLvrCfm : Outport  VectorParamsAs1DForOutWhenUnconnected=off
  wires:
  TrsmNrPreGearAct/1 -> Shift lever confirm logic/3(PreGearRx)
  SftLvrVal/1 -> Shift lever confirm logic/1(ShiftLvrRx)
  TrsmNrGearAct/1 -> Shift lever confirm logic/2(GearRx)
  Shift lever confirm logic/1(SftLvrCfm) -> SftLvrCfm/1

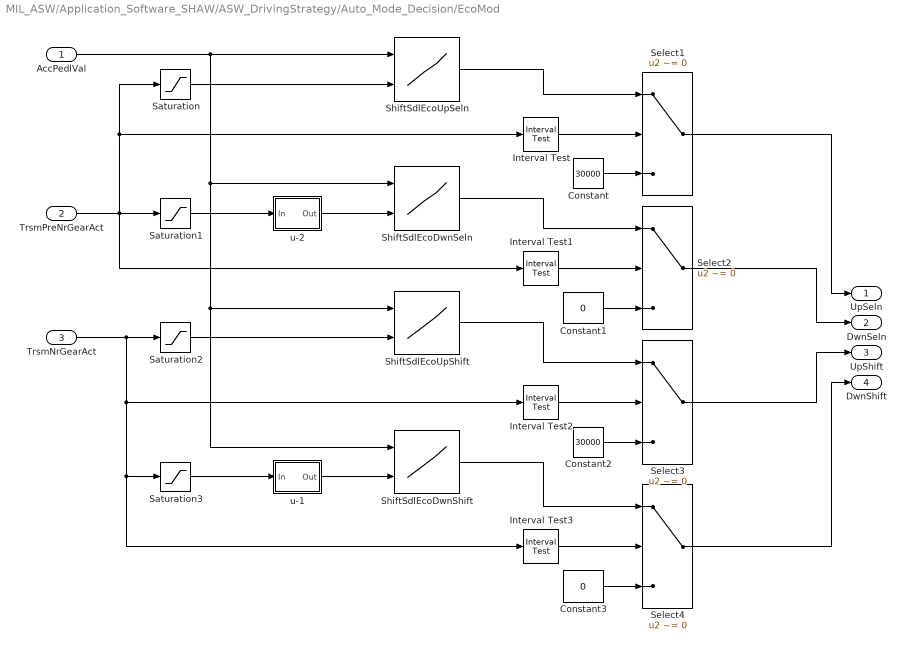
== system MIL_ASW/Application_Software_SHAW/ASW_DrivingStrategy/Auto_Mode_Decision/EcoMod ==
  AccPedlVal : Inport
  TrsmPreNrGearAct : Inport  Port=2
  TrsmNrGearAct : Inport  Port=3
  Constant : Constant  Value=30000  OutDataTypeStr=uint16
  Constant1 : Constant  Value=0  OutDataTypeStr=uint16
  Constant2 : Constant  Value=30000  OutDataTypeStr=uint16
  Constant3 : Constant  Value=0  OutDataTypeStr=uint16
  Interval Test : simulink/Logic and Bit Operations/Interval Test  IntervalClosedRight=on  uplimit=GearMax-1  IntervalClosedLeft=on  lowlimit=1  OutDataTypeStr=uint8
  Interval Test1 : simulink/Logic and Bit Operations/Interval Test  IntervalClosedRight=on  uplimit=GearMax  IntervalClosedLeft=on  lowlimit=2  OutDataTypeStr=uint8
  Interval Test2 : simulink/Logic and Bit Operations/Interval Test  IntervalClosedRight=on  uplimit=GearMax-1  IntervalClosedLeft=on  lowlimit=1  OutDataTypeStr=uint8
  Interval Test3 : simulink/Logic and Bit Operations/Interval Test  IntervalClosedRight=on  uplimit=GearMax  IntervalClosedLeft=on  lowlimit=2  OutDataTypeStr=uint8
  Saturation : Saturate  UpperLimit=GearMax-1  LowerLimit=1  OutDataTypeStr=uint8
  Saturation1 : Saturate  UpperLimit=GearMax  LowerLimit=2  OutDataTypeStr=uint8
  Saturation2 : Saturate  UpperLimit=GearMax-1  LowerLimit=1  OutDataTypeStr=uint8
  Saturation3 : Saturate  UpperLimit=GearMax  LowerLimit=2  OutDataTypeStr=uint8
  Select{1..4} (4 alike) : Switch  Criteria=u2 ~= 0
  ShiftSdlEcoDwnSeln : Lookup_n-D  BreakpointsForDimension1=ShiftSdlThrPedlIdx  BreakpointsForDimension2=GearIdx  Table=ShiftSdlEcoDwnSeln  TableDataTypeStr=uint16  ExtrapMethod=Clip  OutDataTypeStr=Inherit: Inherit from 'Table data'  RndMeth=Simplest  InputSameDT=on
  ShiftSdlEcoDwnShift : Lookup_n-D  BreakpointsForDimension1=ShiftSdlThrPedlIdx  BreakpointsForDimension2=GearIdx  Table=ShiftSdlEcoDwnShift  TableDataTypeStr=uint16  ExtrapMethod=Clip  OutDataTypeStr=Inherit: Inherit from 'Table data'  RndMeth=Simplest  InputSameDT=on
  ShiftSdlEcoUpSeln : Lookup_n-D  BreakpointsForDimension1=ShiftSdlThrPedlIdx  BreakpointsForDimension2=GearIdx  Table=ShiftSdlEcoUpSeln  TableDataTypeStr=uint16  ExtrapMethod=Clip  OutDataTypeStr=Inherit: Inherit from 'Table data'  RndMeth=Simplest  InputSameDT=on
  ShiftSdlEcoUpShift : Lookup_n-D  BreakpointsForDimension1=ShiftSdlThrPedlIdx  BreakpointsForDimension2=GearIdx  Table=ShiftSdlEcoUpShift  TableDataTypeStr=uint16  ExtrapMethod=Clip  OutDataTypeStr=Inherit: Inherit from 'Table data'  RndMeth=Simplest  InputSameDT=on
  u-1 : Subsystem
  u-2 : Subsystem
  UpSeln : Outport  VectorParamsAs1DForOutWhenUnconnected=off
  DwnSeln : Outport  Port=2  VectorParamsAs1DForOutWhenUnconnected=off
  UpShift : Outport  Port=3  VectorParamsAs1DForOutWhenUnconnected=off
  DwnShift : Outport  Port=4  VectorParamsAs1DForOutWhenUnconnected=off
  wires:
  TrsmNrGearAct/1 -> Saturation2/1, Interval Test3/1, Saturation3/1, Interval Test2/1
  Saturation3/1 -> u-1/1(In)
  Saturation1/1 -> u-2/1(In)
  Saturation2/1 -> ShiftSdlEcoUpShift/2
  Saturation/1 -> ShiftSdlEcoUpSeln/2
  Select4/1 -> DwnShift/1
  Select3/1 -> UpShift/1
  Select2/1 -> DwnSeln/1
  Select1/1 -> UpSeln/1
  Constant3/1 -> Select4/3
  Constant2/1 -> Select3/3
  Constant1/1 -> Select2/3
  Constant/1 -> Select1/3
  Interval Test3/1 -> Select4/2
  Interval Test2/1 -> Select3/2
  Interval Test1/1 -> Select2/2
  Interval Test/1 -> Select1/2
  ShiftSdlEcoDwnShift/1 -> Select4/1
  ShiftSdlEcoUpShift/1 -> Select3/1
  ShiftSdlEcoDwnSeln/1 -> Select2/1
  ShiftSdlEcoUpSeln/1 -> Select1/1
  AccPedlVal/1 -> ShiftSdlEcoUpSeln/1, ShiftSdlEcoDwnShift/1, ShiftSdlEcoUpShift/1, ShiftSdlEcoDwnSeln/1
  u-2/1(Out) -> ShiftSdlEcoDwnSeln/2
  u-1/1(Out) -> ShiftSdlEcoDwnShift/2
  TrsmPreNrGearAct/1 -> Interval Test1/1, Saturation1/1, Interval Test/1, Saturation/1

== system MIL_ASW/Application_Software_SHAW/ASW_DrivingStrategy/Auto_Mode_Decision/Eco_Spt_Schedule_Mix ==
  DrvrInten : Inport
  EcoShiftSpd : Inport  Port=2
  SptShiftSpd : Inport  Port=3
  Add : Sum  AccumDataTypeStr=uint16
  Constant : Constant  Value=75  OutDataTypeStr=int16
  Constant1 : Constant  Value=25  OutDataTypeStr=int16
  Data Type Conversion : DataTypeConversion  OutDataTypeStr=int16
  Data Type Conversion1 : DataTypeConversion  OutDataTypeStr=int16
  Divide : Product  Inputs=*/  OutDataTypeStr=Inherit: Same as first input
  Gain : Gain  Gain=100  OutDataTypeStr=Inherit: Same as input
  Gain1 : Gain  Gain=1/100  OutDataTypeStr=Inherit: Same as input
  Product : Product  OutDataTypeStr=int32
  Saturation Dynamic : simulink/Discontinuities/Saturation Dynamic  OutMin=[]  OutMax=[]  OutDataTypeStr=Inherit: Same as second input  OutDataType=fixdt(1, 16)  OutScaling=2^-10  DoSatur=off
  Scope{1..5} (5 alike) : Scope
  Subtract : Sum  Inputs=+-
  Subtract1 : Sum  Inputs=+-
  Subtract2 : Sum  Inputs=+-  OutDataTypeStr=int16
  MixShiftSpd : Outport  VectorParamsAs1DForOutWhenUnconnected=off
  wires:
  DrvrInten/1 -> Saturation Dynamic/2
  Constant/1 -> Subtract1/1, Saturation Dynamic/1
  Constant1/1 -> Subtract1/2, Subtract/2, Saturation Dynamic/3
  Saturation Dynamic/1 -> Subtract/1
  Subtract/1 -> Gain/1
  SptShiftSpd/1 -> Data Type Conversion/1
  Gain/1 -> Divide/1
  Subtract1/1 -> Divide/2
  Divide/1 -> Scope4/1, Product/1
  Subtract2/1 -> Scope5/1, Product/2
  Product/1 -> Gain1/1
  Gain1/1 -> Add/1
  Add/1 -> Scope1/1, MixShiftSpd/1
  EcoShiftSpd/1 -> Data Type Conversion1/1
  Data Type Conversion/1 -> Scope2/1, Subtract2/1
  Data Type Conversion1/1 -> Scope3/1, Subtract2/2, Add/2

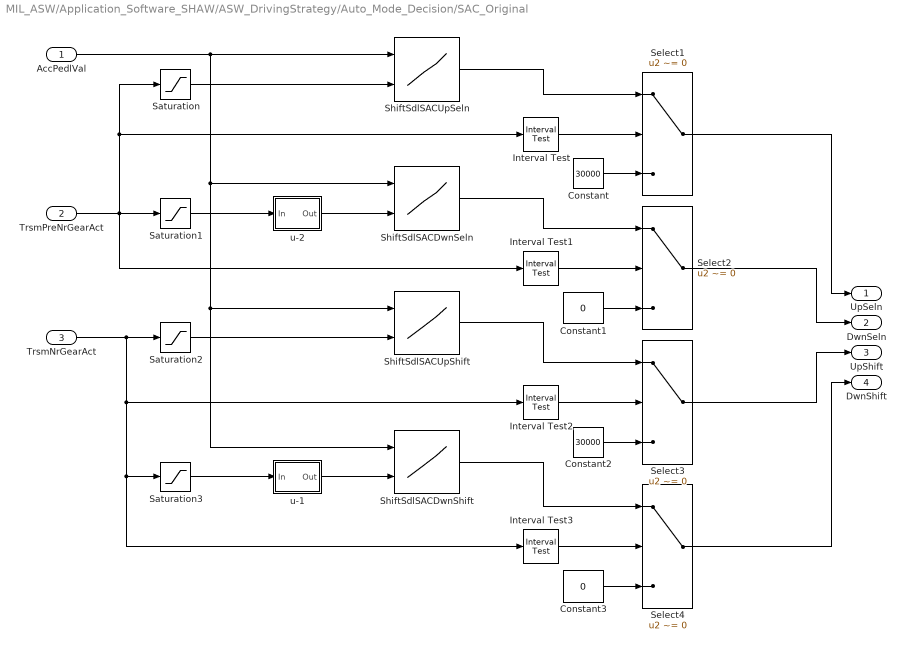
== system MIL_ASW/Application_Software_SHAW/ASW_DrivingStrategy/Auto_Mode_Decision/SAC_Original ==
  AccPedlVal : Inport
  TrsmPreNrGearAct : Inport  Port=2
  TrsmNrGearAct : Inport  Port=3
  Constant : Constant  Value=30000  OutDataTypeStr=uint16
  Constant1 : Constant  Value=0  OutDataTypeStr=uint16
  Constant2 : Constant  Value=30000  OutDataTypeStr=uint16
  Constant3 : Constant  Value=0  OutDataTypeStr=uint16
  Interval Test : simulink/Logic and Bit Operations/Interval Test  IntervalClosedRight=on  uplimit=GearMax-1  IntervalClosedLeft=on  lowlimit=1  OutDataTypeStr=uint8
  Interval Test1 : simulink/Logic and Bit Operations/Interval Test  IntervalClosedRight=on  uplimit=GearMax  IntervalClosedLeft=on  lowlimit=2  OutDataTypeStr=uint8
  Interval Test2 : simulink/Logic and Bit Operations/Interval Test  IntervalClosedRight=on  uplimit=GearMax-1  IntervalClosedLeft=on  lowlimit=1  OutDataTypeStr=uint8
  Interval Test3 : simulink/Logic and Bit Operations/Interval Test  IntervalClosedRight=on  uplimit=GearMax  IntervalClosedLeft=on  lowlimit=2  OutDataTypeStr=uint8
  Saturation : Saturate  UpperLimit=GearMax-1  LowerLimit=1  OutDataTypeStr=uint8
  Saturation1 : Saturate  UpperLimit=GearMax  LowerLimit=2  OutDataTypeStr=uint8
  Saturation2 : Saturate  UpperLimit=GearMax-1  LowerLimit=1  OutDataTypeStr=uint8
  Saturation3 : Saturate  UpperLimit=GearMax  LowerLimit=2  OutDataTypeStr=uint8
  Select{1..4} (4 alike) : Switch  Criteria=u2 ~= 0
  ShiftSdlSACDwnSeln : Lookup_n-D  BreakpointsForDimension1=ShiftSdlThrPedlIdx  BreakpointsForDimension2=GearIdx  Table=ShiftSdlSACDwnSeln  TableDataTypeStr=uint16  ExtrapMethod=Clip  OutDataTypeStr=Inherit: Inherit from 'Table data'  RndMeth=Simplest  InputSameDT=on
  ShiftSdlSACDwnShift : Lookup_n-D  BreakpointsForDimension1=ShiftSdlThrPedlIdx  BreakpointsForDimension2=GearIdx  Table=ShiftSdlSACDwnShift  TableDataTypeStr=uint16  ExtrapMethod=Clip  OutDataTypeStr=Inherit: Inherit from 'Table data'  RndMeth=Simplest  InputSameDT=on
  ShiftSdlSACUpSeln : Lookup_n-D  BreakpointsForDimension1=ShiftSdlThrPedlIdx  BreakpointsForDimension2=GearIdx  Table=ShiftSdlSACUpSeln  TableDataTypeStr=uint16  ExtrapMethod=Clip  OutDataTypeStr=Inherit: Inherit from 'Table data'  RndMeth=Simplest  InputSameDT=on
  ShiftSdlSACUpShift : Lookup_n-D  BreakpointsForDimension1=ShiftSdlThrPedlIdx  BreakpointsForDimension2=GearIdx  Table=ShiftSdlSACUpShift  TableDataTypeStr=uint16  ExtrapMethod=Clip  OutDataTypeStr=Inherit: Inherit from 'Table data'  RndMeth=Simplest  InputSameDT=on
  u-1 : Subsystem
  u-2 : Subsystem
  UpSeln : Outport  VectorParamsAs1DForOutWhenUnconnected=off
  DwnSeln : Outport  Port=2  VectorParamsAs1DForOutWhenUnconnected=off
  UpShift : Outport  Port=3  VectorParamsAs1DForOutWhenUnconnected=off
  DwnShift : Outport  Port=4  VectorParamsAs1DForOutWhenUnconnected=off
  wires:
  TrsmNrGearAct/1 -> Saturation2/1, Interval Test3/1, Saturation3/1, Interval Test2/1
  Saturation3/1 -> u-1/1(In)
  Saturation1/1 -> u-2/1(In)
  Saturation2/1 -> ShiftSdlSACUpShift/2
  Saturation/1 -> ShiftSdlSACUpSeln/2
  Select4/1 -> DwnShift/1
  Select3/1 -> UpShift/1
  Select2/1 -> DwnSeln/1
  Select1/1 -> UpSeln/1
  Constant3/1 -> Select4/3
  Constant2/1 -> Select3/3
  Constant1/1 -> Select2/3
  Constant/1 -> Select1/3
  Interval Test3/1 -> Select4/2
  Interval Test2/1 -> Select3/2
  Interval Test1/1 -> Select2/2
  Interval Test/1 -> Select1/2
  ShiftSdlSACDwnShift/1 -> Select4/1
  ShiftSdlSACUpShift/1 -> Select3/1
  ShiftSdlSACDwnSeln/1 -> Select2/1
  ShiftSdlSACUpSeln/1 -> Select1/1
  AccPedlVal/1 -> ShiftSdlSACUpSeln/1, ShiftSdlSACDwnShift/1, ShiftSdlSACUpShift/1, ShiftSdlSACDwnSeln/1
  u-2/1(Out) -> ShiftSdlSACDwnSeln/2
  u-1/1(Out) -> ShiftSdlSACDwnShift/2
  TrsmPreNrGearAct/1 -> Interval Test1/1, Saturation1/1, Interval Test/1, Saturation/1
